simulink model "disturbances_report_sim"  (R2023b)
settings: Solver=ode5  StartTime=0.0  StopTime=5643.69  FixedStep=1  RelTol=1e-3
values from neighbouring files (symbols this model uses):
  A = [0.49 0.49 0.49 0.49 0.49 0.49 0.49 0.49 0.49 0.49 0.49 0.49 0.49 0.49]    [disturbances_report.m]    (also in sat_dist.m = [6*1e-2; 6*1e-2; 6*1e-2; 6*1e-2; 4*1e-2; 4*1e-2; 12*1e-2; 12)
  a = 1 / ( (2/r) - (v^2 / mu) )    [car2par.m]    (also in disturbances_report.m = 6851.22197053)
  c1 = [1 - rho_s; 1 - rho_s; 1 - rho_s]    [disturbances_report.m]
  CD = 2.2    [disturbances_report.m]
  d0 = 1.585*10^-12    (= 1.585e-12)    [disturbances_report.m]
  e = norm(ee)    [car2par.m]    (also in disturbances_report.m = 0.00183012221618)
  H = 60.828    [disturbances_report.m]
  h0 = 450    [disturbances_report.m]
  i = rad2deg(i)    [car2par.m]    (also in disturbances_report.m = 1.69998086203)
  I_ext = diag([I1_ext I2_ext I3_ext])    [disturbances_report.m]
  Iinv_ext = I_ext\eye(3)    [disturbances_report.m]
  jb = [0.01; 0.05; 0.01]    [disturbances_report.m]    (also in sat_dist.m)
  muE = astroConstants(13)    [disturbances_report.m]
  N = [1 0 0]'    [car2par.m]    (also in disturbances_report.m = [0 1 0; 0 -1 0; sqrt(2)/2 0 sqrt(2)/2; -sqrt(2)/2 0 sqrt(2)/; sat_dist.m = [1 0 0; 0 1 0; -1 0 0; 0 -1 0; 0 0 1; 0 0 -1; 1 0 0; -1 0 0;)
  n_sun = sqrt(mu_sun/a_E^3)    [disturbances_report.m]
  nn = sqrt(muE/a^3)    [disturbances_report.m]
  om = rad2deg(om)    [car2par.m]    (also in disturbances_report.m = 1.77284810319)
  OM = rad2deg(OM)    [car2par.m]    (also in disturbances_report.m = 0.55426850949)
  omega0 = zeros(3,1)    [disturbances_report.m]    (also in sat_dist.m = [0; 0; n])
  omegaE = deg2rad(15)/3600    [disturbances_report.m]    (also in sat_dist.m)
  onesM = ones(3, n)    [disturbances_report.m]
  onesV = ones(n,1)    [disturbances_report.m]
  P = astroConstants(31)/(astroConstants(5)*10^3)    [disturbances_report.m]    (also in sat_dist.m = Fe/c)
  r_Fskew = zeros(n*3, n*3)    [disturbances_report.m]
  rho_d = [0.1 0.1 0.1 0.1 0.1 0.1 0.1 0.1 0.1 0.1 0.1 0.1 0.1 0.1]    [disturbances_report.m]
  rho_s = [0.5 0.5 0.5 0.5 0.5 0.5 0.1 0.1 0.1 0.1 0.1 0.1 0.1 0.1]    [disturbances_report.m]
  Rt = astroConstants(23)    [disturbances_report.m]    (also in sat_dist.m)
  s0 = zeros(3,1)    [disturbances_report.m]    (also in sat_dist.m)
  th_0 = 0    [disturbances_report.m]
  tol = 0.2    [disturbances_report.m]
undefined symbols (not defined in the file or in its folder): gh, magnitude
libraries: matrix_library x6, simulink x4, simulink_extras x1, dspmathops x1
(part 1 of 2)
settings Model: Creator=danie  LastModifiedBy=danie

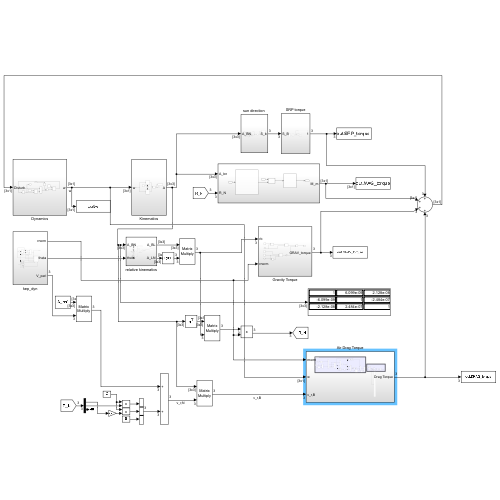
[thumbnail: Simulink's stored preview of the top-level diagram]
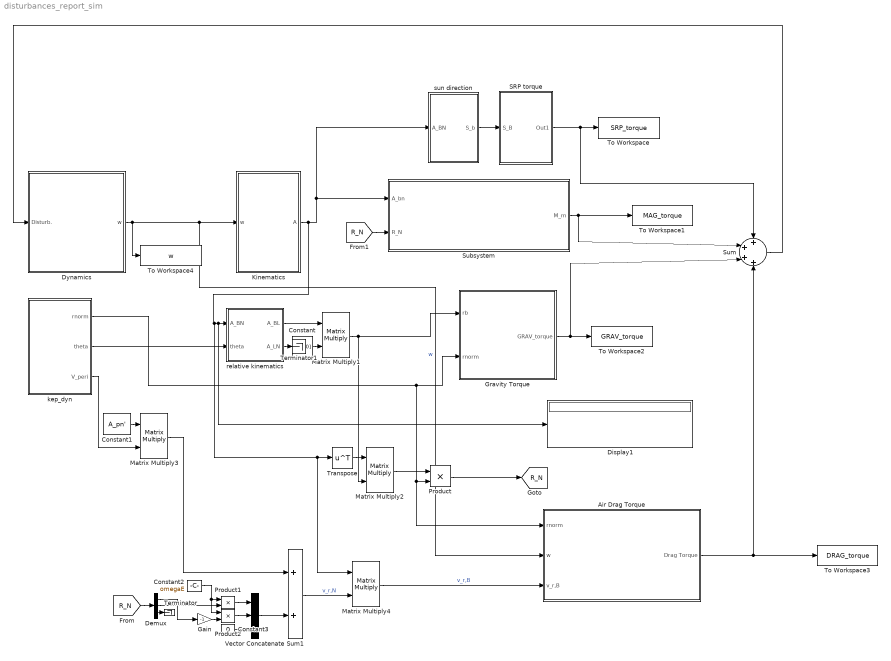
== system disturbances_report_sim ==
  Air Drag Torque : Subsystem
  Constant : Constant  Value=[1;0;0]
  Constant1 : Constant  Value=A_pn'
  Constant2 : Constant  Value=omegaE
  Constant3 : Constant  Value=0
  Demux : Demux  Outputs=3
  Display1 : Display
  Dynamics : Subsystem
  Gain : Gain  Gain=-1
  Gravity Torque : Subsystem
  Kinematics : Subsystem
  Matrix Multiply{1..4} (4 alike) : Product  Multiplication=Matrix(*)
  Product : Product
  Product1 : Product
  Product2 : Product
  SRP torque : Subsystem
  Subsystem : Subsystem
  Sum : Sum  Inputs=++++
  Sum1 : Sum
  Terminator : Terminator
  Terminator1 : Terminator
  To Workspace : ToWorkspace  VariableName=SRP_torque  SaveFormat=Timeseries  SampleTime=-1
  To Workspace1 : ToWorkspace  VariableName=MAG_torque  SampleTime=-1
  To Workspace2 : ToWorkspace  VariableName=GRAV_torque  SaveFormat=Timeseries  SampleTime=-1
  To Workspace3 : ToWorkspace  VariableName=DRAG_torque  SaveFormat=Timeseries  SampleTime=-1
  To Workspace4 : ToWorkspace  VariableName=w  SaveFormat=Timeseries  SampleTime=-1
  Transpose : Math  Operator=transpose
  Vector Concatenate : Concatenate  NumInputs=3
  kep_dyn : Subsystem
  relative kinematics : Subsystem
  "sun direction " : Subsystem
  tag scope: R_N=global
  wires:
  Dynamics/1(w) -> To Workspace4/1, Kinematics/1(w), Air Drag Torque/2(w)  "w"
  kep_dyn/2(theta) -> relative kinematics/2(theta)
  Kinematics/1(A) -> Subsystem/1(A_bn), "sun direction "/1(A_BN), Matrix Multiply4/1, Transpose/1, Display1/1, relative kinematics/1(A_BN)
  SRP torque/1(Out1) -> Sum/1, To Workspace/1
  Matrix Multiply1/1 -> Gravity Torque/1(rb), Matrix Multiply2/2
  Gravity Torque/1(GRAV_torque) -> Sum/3, To Workspace2/1
  relative kinematics/1(A_BL) -> Matrix Multiply1/1
  relative kinematics/2(A_LN) -> Terminator1/1
  "sun direction "/1(S_b) -> SRP torque/1(S_B)
  Sum/1 -> Dynamics/1(Disturb.)
  Constant/1 -> Matrix Multiply1/2
  kep_dyn/1(rnorm) -> Air Drag Torque/1(rnorm), Product/2, Gravity Torque/2(rnorm)
  Transpose/1 -> Matrix Multiply2/1
  Matrix Multiply2/1 -> Product/1
  kep_dyn/3(V_peri) -> Matrix Multiply3/2
  Constant1/1 -> Matrix Multiply3/1
  Matrix Multiply3/1 -> Sum1/1
  Vector Concatenate/1 -> Sum1/2
  Constant3/1 -> Vector Concatenate/3
  Product2/1 -> Vector Concatenate/2
  Product1/1 -> Vector Concatenate/1
  Constant2/1 -> Product2/1, Product1/1
  Product/1 -> [R_N]
  [R_N] -> Demux/1
  Demux/2 -> Product1/2
  Demux/1 -> Gain/1
  Gain/1 -> Product2/2
  Demux/3 -> Terminator/1
  Sum1/1 -> Matrix Multiply4/2  "v_r,N"
  Matrix Multiply4/1 -> Air Drag Torque/3(v_r,B)  "v_r,B"
  Air Drag Torque/1(Drag Torque) -> To Workspace3/1, Sum/4
  [R_N] -> Subsystem/2(R_N)
  Subsystem/1(M_m) -> Sum/2, To Workspace1/1

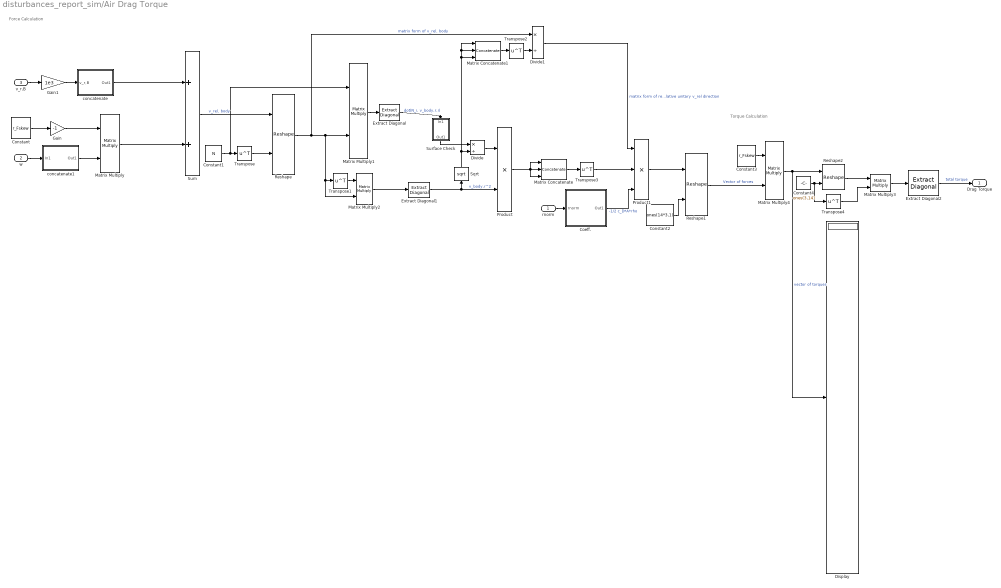
== system disturbances_report_sim/Air Drag Torque ==
  note: Torque Calculation
  note: Force Calculation
  rnorm : Inport
  w : Inport  Port=2
  v_r,B : Inport  Port=3
  Coeff. : Subsystem
  Constant : Constant  Value=r_Fskew
  Constant1 : Constant  Value=N
  Constant2 : Constant  Value=ones(14*3,1)
  Constant3 : Constant  Value=r_Fskew
  Constant4 : Constant  Value=ones(3,14)
  Display : Display
  Divide : Product  Inputs=*/
  Divide1 : Product  Inputs=*/
  Extract Diagonal : matrix_library/Extract Diagonal
      settings: LibrarySourceBlock=|
      | simulink/Matrix
      | Operations/Extract Diagonal
  Extract Diagonal1 : matrix_library/Extract Diagonal
      settings: LibrarySourceBlock=|
      | simulink/Matrix
      | Operations/Extract Diagonal
  Extract Diagonal2 : matrix_library/Extract Diagonal
      settings: LibrarySourceBlock=|
      | simulink/Matrix
      | Operations/Extract Diagonal
  Gain : Gain  Gain=-1
  Gain1 : Gain  Gain=1e3
  Matrix Concatenate : Concatenate  NumInputs=3  Mode=Multidimensional array  ConcatenateDimension=2
  Matrix Concatenate1 : Concatenate  NumInputs=3  Mode=Multidimensional array  ConcatenateDimension=2
  Matrix Multiply{,1..4} (5 alike) : Product  Multiplication=Matrix(*)
  Product : Product
  Product1 : Product  Inputs=3
  Reshape : Reshape  OutputDimensionality=Derive from reference input port
  Reshape1 : Reshape  OutputDimensionality=Derive from reference input port
  Reshape2 : Reshape  OutputDimensionality=Derive from reference input port
  Sqrt : Sqrt
  Sum : Sum
  Surface Check : Subsystem
  Transpose{,1..4} (5 alike) : Math  Operator=transpose
  concatenate : Subsystem
  concatenate1 : Subsystem
  Drag Torque : Outport
  wires:
  Constant/1 -> Gain/1
  Gain/1 -> Matrix Multiply/1
  w/1 -> concatenate1/1(In1)
  concatenate1/1(Out1) -> Matrix Multiply/2
  Matrix Multiply/1 -> Sum/2
  v_r,B/1 -> Gain1/1
  concatenate/1(Out1) -> Sum/1
  Transpose/1 -> Reshape/2
  Constant1/1 -> Matrix Multiply1/1, Transpose/1
  Sum/1 -> Reshape/1  "v_rel, body"
  Reshape/1 -> Transpose1/1, Matrix Multiply2/2, Matrix Multiply1/2, Divide1/1  "matrix form of v_rel, body"
  Matrix Multiply1/1 -> Extract Diagonal/1
  Extract Diagonal/1 -> Surface Check/1(In1)  "dot(N_i, v_body,r,i)"
  Transpose1/1 -> Matrix Multiply2/1
  Matrix Multiply2/1 -> Extract Diagonal1/1
  Extract Diagonal1/1 -> Sqrt/1, Product/2  "v_body,r^2"
  Sqrt/1 -> Divide/2, Matrix Concatenate1/1, Matrix Concatenate1/2, Matrix Concatenate1/3
  Divide/1 -> Product/1
  Product/1 -> Matrix Concatenate/3, Matrix Concatenate/1, Matrix Concatenate/2
  Matrix Concatenate1/1 -> Transpose2/1
  Transpose2/1 -> Divide1/2
  Divide1/1 -> Product1/1  "matrix form of relative unitary v_rel direction"
  Matrix Concatenate/1 -> Transpose3/1
  Surface Check/1(Out1) -> Divide/1
  Coeff./1(Out1) -> Product1/3  "-1/2 c_D*A*rho"
  Transpose3/1 -> Product1/2
  Product1/1 -> Reshape1/1
  Reshape1/1 -> Matrix Multiply4/2  "Vector of forces"
  Constant2/1 -> Reshape1/2
  Constant3/1 -> Matrix Multiply4/1
  Matrix Multiply4/1 -> Display/1, Reshape2/1  "vector of torques"
  rnorm/1 -> Coeff./1(rnorm)
  Constant4/1 -> Transpose4/1, Reshape2/2
  Reshape2/1 -> Matrix Multiply3/1
  Transpose4/1 -> Matrix Multiply3/2
  Matrix Multiply3/1 -> Extract Diagonal2/1
  Extract Diagonal2/1 -> Drag Torque/1  "total torque"
  Gain1/1 -> concatenate/1(v_r,B)

== system disturbances_report_sim/Dynamics ==
  Disturb. : Inport
  Constant : Constant  Value=I_ext
  Constant1 : Constant  Value=Iinv_ext
  Cross Product : matrix_library/Cross Product
  Integrator : Integrator  InitialCondition=omega0
  Product : Product  Multiplication=Matrix(*)
  Product1 : Product  Multiplication=Matrix(*)
  Reshape : Reshape  OutputDimensionality=Column vector (2-D)
  Sum : Sum  Inputs=+-
  w : Outport
  wires:
  Constant/1 -> Product/1
  Integrator/1 -> w/1, Cross Product/1, Product/2  "w"
  Constant1/1 -> Product1/1
  Product/1 -> Cross Product/2
  Product1/1 -> Integrator/1  "wdot"
  Disturb./1 -> Reshape/1
  Sum/1 -> Product1/2
  Cross Product/1 -> Sum/2
  Reshape/1 -> Sum/1

== system disturbances_report_sim/Gravity Torque ==
  rb : Inport
  rnorm : Inport  Port=2
  Constant : Constant  Value=muE
  Constant1 : Constant  Value=I_ext
  Constant3 : Constant  Value=3
  Cross Product : matrix_library/Cross Product
  Divide : Product  Inputs=**/
  Gain : Gain  Gain=-1
  Matrix Multiply : Product  Multiplication=Matrix(*)
  Power : Math  Operator=pow
  Product : Product
  GRAV_torque : Outport
  wires:
  Constant1/1 -> Matrix Multiply/1
  rb/1 -> Matrix Multiply/2, Cross Product/2
  Matrix Multiply/1 -> Cross Product/1
  Constant3/1 -> Power/2, Divide/2
  Power/1 -> Divide/3
  Constant/1 -> Divide/1
  Divide/1 -> Gain/1
  Gain/1 -> Product/2
  Cross Product/1 -> Product/1
  Product/1 -> GRAV_torque/1
  rnorm/1 -> Power/1

== system disturbances_report_sim/Kinematics ==
  w : Inport
  Kinematics 312 : Subsystem
  Kinematics 313 : Subsystem
  Merge : Merge
  NOT : Logic  Operator=NOT  IconShape=distinctive  AllPortsSameDT=off  OutDataTypeStr=boolean
  System switcher : Subsystem
  To Workspace : ToWorkspace  VariableName=A  SaveFormat=Timeseries  SampleTime=-1
  A : Outport
  wires:
  NOT/1 -> Kinematics 313/Enable
  w/1 -> Kinematics 312/1(w), Kinematics 313/1(w)
  System switcher/1(flag) -> Kinematics 312/Enable, NOT/1
  Kinematics 313/1(A) -> Merge/2
  Merge/1 -> A/1, To Workspace/1  "A"
  Kinematics 312/1(A) -> Merge/1

== system disturbances_report_sim/SRP torque ==
  S_B : Inport
  Display : Display
  SRP forces calc : Subsystem
  To Workspace : ToWorkspace  VariableName=SRP_F  SaveFormat=Timeseries  SampleTime=-1
  To Workspace1 : ToWorkspace  VariableName=SRP_T  SaveFormat=Timeseries  SampleTime=-1
  equivalent force system : Subsystem
  Out1 : Outport
  wires:
  equivalent force system/1(Torque) -> Display/1, To Workspace1/1, Out1/1
  equivalent force system/2(Resultant) -> To Workspace/1
  S_B/1 -> SRP forces calc/1(In1)  "SUN DIR."
  SRP forces calc/1(forces) -> equivalent force system/1(Forces)

== system disturbances_report_sim/Subsystem ==
  A_bn : Inport
  R_N : Inport  Port=2
  Magnetic Field : Subsystem
  Magnetic Torque 1 : Subsystem
  Matrix Multiply : Product  Multiplication=Matrix(*)
  M_m : Outport
  wires:
  Magnetic Field/1(B_N) -> Matrix Multiply/2
  Matrix Multiply/1 -> Magnetic Torque 1/1(B_b)
  R_N/1 -> Magnetic Field/1(R_N)
  Magnetic Torque 1/1(M_m) -> M_m/1
  A_bn/1 -> Matrix Multiply/1

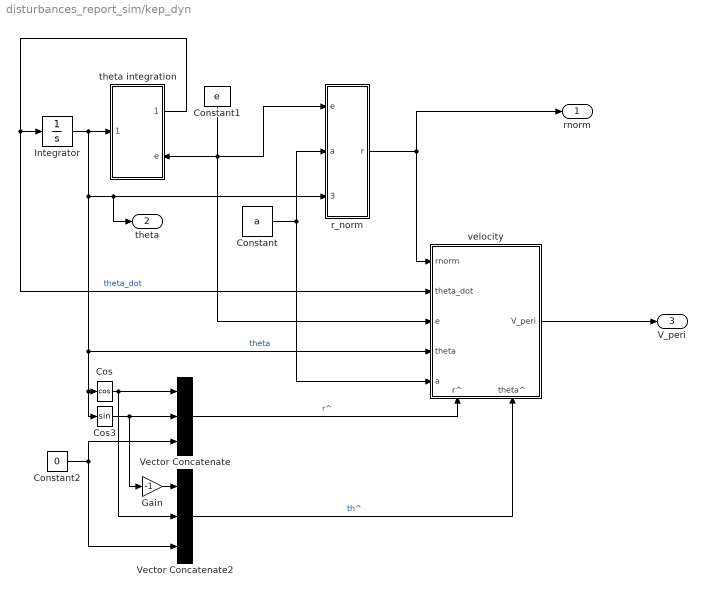
== system disturbances_report_sim/kep_dyn ==
  Constant : Constant  Value=a
  Constant1 : Constant  Value=e
  Constant2 : Constant  Value=0
  Cos : Trigonometry  Operator=cos
  Cos3 : Trigonometry
  Gain : Gain  Gain=-1
  Integrator : Integrator  InitialCondition=th_0
  Vector Concatenate : Concatenate  NumInputs=3
  Vector Concatenate2 : Concatenate  NumInputs=3
  r_norm : Subsystem
  theta integration : Subsystem
      settings: PortSchema="{\"entries\":[{\"content\":{\"sides\":[{\"content\":{\"connectorIds\":[\"In1\"]},\"type\":\"ConnectorPlacement.EquallySpacedRectSide\",\"uuid\":\"3f1b1ec9-07ed-4eb1-9e41-630dc5613e97\"},{\"content\":{\"connectorIds\":[\"Out1\",\"In2\"],\"side\":\"RIGHT\"},\"type\":\"ConnectorPlacement.EquallySpacedRectSide\",\"uuid\":\"22d0f7bc-714c-4365-a26c-07047ff4be14\"},{\"content\":{\"side\":\"TOP\"},\"type\":\"ConnectorPlacement.EquallySpacedRectSide\",\"uuid\":\"875f7006-d698-4730-93ae-1a7d05f24054\"}]},\"type\":\"ConnectorPlacement.EquallySpacedConnector\",\"uuid\":\"799b65b1-faea-432b-9f3f-2d21984184cd\"}],\"packageUris\":[\"http://schema.mathworks.com/mf0/Connector/R2020b\"],\"version\":\"1.0\"}"
  velocity : Subsystem
      settings: PortSchema="{\"entries\":[{\"content\":{\"sides\":[{\"content\":{\"connectorIds\":[\"In1\",\"In2\",\"In3\",\"In4\",\"In5\"]},\"type\":\"ConnectorPlacement.EquallySpacedRectSide\",\"uuid\":\"462ea4ff-c936-4e9a-a15d-c684549947ff\"},{\"content\":{\"connectorIds\":[\"Out1\"],\"side\":\"RIGHT\"},\"type\":\"ConnectorPlacement.EquallySpacedRectSide\",\"uuid\":\"a4e336f6-8704-425f-b778-b72f089cf101\"},{\"content\":{\"side\":\"TOP\"},\"type\":\"ConnectorPlacement.EquallySpacedRectSide\",\"uuid\":\"dc4110a0-1fc3-4f7c-9a82-d4e052a3954d\"},{\"content\":{\"connectorIds\":[\"In6\",\"In7\"],\"side\":\"BOTTOM\"},\"type\":\"ConnectorPlacement.EquallySpacedRectSide\",\"uuid\":\"58c8717a-d2ad-44bd-b5d0-69e581fda9fe\"}]},\"type\":\"ConnectorPlacement.EquallySpacedConnector\",\"uuid\":\"b458c0bc-27e5-4a27-9089-a782da5757b6\"}],\"packageUris\":[\"http://schema.mathworks.com/mf0/Connector/R2020b\"],\"version\":\"1.0\"}"
  rnorm : Outport
  theta : Outport  Port=2
  V_peri : Outport  Port=3
  wires:
  Integrator/1 -> Cos3/1, Cos/1, velocity/4(theta), theta/1, r_norm/3(theta), theta integration/1(theta)  "theta"
  theta integration/1(theta_dot) -> velocity/2(theta_dot), Integrator/1  "theta_dot"
  Constant1/1 -> r_norm/1(e), theta integration/2(e), velocity/3(e)
  r_norm/1(r) -> velocity/1(rnorm), rnorm/1
  Constant/1 -> velocity/5(a), r_norm/2(a)
  Cos/1 -> Vector Concatenate2/2, Vector Concatenate/1
  Cos3/1 -> Gain/1, Vector Concatenate/2
  Constant2/1 -> Vector Concatenate/3, Vector Concatenate2/3
  Gain/1 -> Vector Concatenate2/1
  Vector Concatenate/1 -> velocity/6(r^)  "r^"
  Vector Concatenate2/1 -> velocity/7(theta^)  "th^"
  velocity/1(V_peri) -> V_peri/1

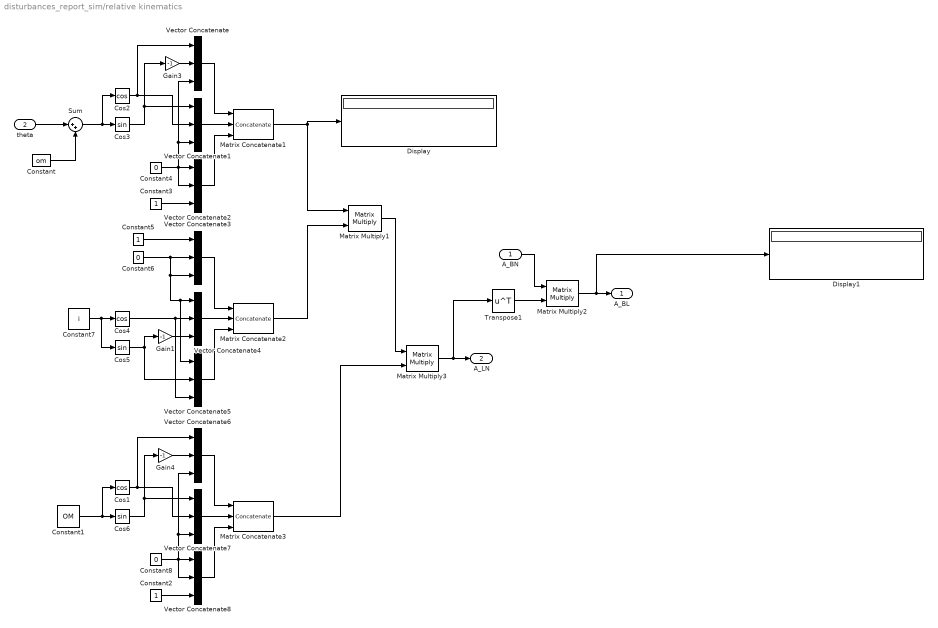
== system disturbances_report_sim/relative kinematics ==
  A_BN : Inport
  theta : Inport  Port=2
  Constant : Constant  Value=om
  Constant1 : Constant  Value=OM
  Constant2 : Constant
  Constant3 : Constant
  Constant4 : Constant  Value=0
  Constant5 : Constant
  Constant6 : Constant  Value=0
  Constant7 : Constant  Value=i
  Constant8 : Constant  Value=0
  Cos1 : Trigonometry  Operator=cos
  Cos2 : Trigonometry  Operator=cos
  Cos3 : Trigonometry
  Cos4 : Trigonometry  Operator=cos
  Cos5 : Trigonometry
  Cos6 : Trigonometry
  Display : Display
  Display1 : Display
  Gain1 : Gain  Gain=-1
  Gain3 : Gain  Gain=-1
  Gain4 : Gain  Gain=-1
  Matrix Concatenate1 : Concatenate  NumInputs=3  Mode=Multidimensional array  ConcatenateDimension=2
  Matrix Concatenate2 : Concatenate  NumInputs=3  Mode=Multidimensional array  ConcatenateDimension=2
  Matrix Concatenate3 : Concatenate  NumInputs=3  Mode=Multidimensional array  ConcatenateDimension=2
  Matrix Multiply1 : Product  Multiplication=Matrix(*)
  Matrix Multiply2 : Product  Multiplication=Matrix(*)
  Matrix Multiply3 : Product  Multiplication=Matrix(*)
  Sum : Sum  Inputs=|++
  Transpose1 : Math  Operator=transpose
  Vector Concatenate{,1..8} (9 alike) : Concatenate  NumInputs=3
  A_BL : Outport
  A_LN : Outport  Port=2
  wires:
  Cos2/1 -> Vector Concatenate1/2, Vector Concatenate/1
  Constant4/1 -> Vector Concatenate2/2, Vector Concatenate/3, Vector Concatenate1/3, Vector Concatenate2/1
  Constant3/1 -> Vector Concatenate2/3
  Cos3/1 -> Vector Concatenate1/1, Gain3/1
  Vector Concatenate/1 -> Matrix Concatenate1/1
  Vector Concatenate1/1 -> Matrix Concatenate1/2
  Vector Concatenate2/1 -> Matrix Concatenate1/3
  Vector Concatenate5/1 -> Matrix Concatenate2/3
  Constant7/1 -> Cos4/1, Cos5/1
  Vector Concatenate3/1 -> Matrix Concatenate2/1
  Vector Concatenate4/1 -> Matrix Concatenate2/2
  Constant5/1 -> Vector Concatenate3/1
  Constant6/1 -> Vector Concatenate5/1, Vector Concatenate4/1, Vector Concatenate3/3, Vector Concatenate3/2
  Cos4/1 -> Vector Concatenate4/2, Vector Concatenate5/3
  Cos5/1 -> Vector Concatenate5/2, Gain1/1
  Matrix Concatenate1/1 -> Matrix Multiply1/1, Display/1
  Matrix Concatenate2/1 -> Matrix Multiply1/2
  Matrix Multiply1/1 -> Matrix Multiply3/1
  A_BN/1 -> Matrix Multiply2/1
  Transpose1/1 -> Matrix Multiply2/2
  Matrix Multiply2/1 -> Display1/1, A_BL/1
  Constant/1 -> Sum/2
  theta/1 -> Sum/1
  Sum/1 -> Cos2/1, Cos3/1
  Constant8/1 -> Vector Concatenate8/2, Vector Concatenate6/3, Vector Concatenate7/3, Vector Concatenate8/1
  Vector Concatenate7/1 -> Matrix Concatenate3/2
  Vector Concatenate6/1 -> Matrix Concatenate3/1
  Vector Concatenate8/1 -> Matrix Concatenate3/3
  Matrix Concatenate3/1 -> Matrix Multiply3/2
  Cos1/1 -> Vector Concatenate7/2, Vector Concatenate6/1
  Constant2/1 -> Vector Concatenate8/3
  Cos6/1 -> Vector Concatenate7/1, Gain4/1
  Constant1/1 -> Cos1/1, Cos6/1
  Matrix Multiply3/1 -> Transpose1/1, A_LN/1
  Gain3/1 -> Vector Concatenate/2
  Gain4/1 -> Vector Concatenate6/2
  Gain1/1 -> Vector Concatenate4/3

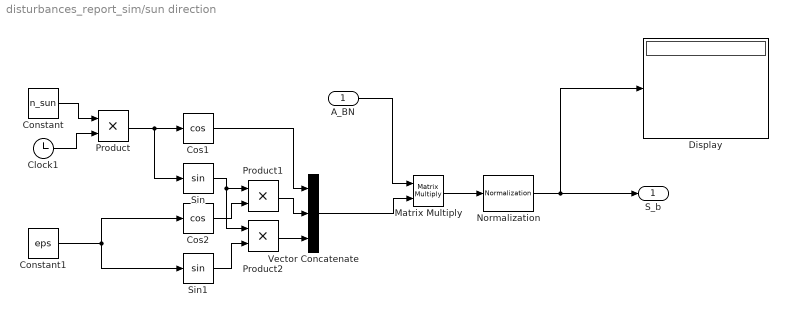
== system disturbances_report_sim/sun direction  ==
  A_BN : Inport
  Clock1 : Clock
  Constant : Constant  Value=n_sun
  Constant1 : Constant  Value=eps
  Cos1 : Trigonometry  Operator=cos
  Cos2 : Trigonometry  Operator=cos
  Display : Display
  Matrix Multiply : Product  Multiplication=Matrix(*)
  Normalization : dspmathops/Normalization  NormType=Squared 2-norm  Bias=1e-10  NormOver=Each column  Dimension=1  roundingMode=Floor  overflowMode=off  accumDataTypeStr=Inherit: Same as product output  accumLastDataTypeStr=Inherit: Same as product output  outputDataTypeStr=Inherit: Same as product output  outputMin=[]  outputMax=[]  outputLastDataTypeStr=Inherit: Same as product output
  Product : Product
  Product1 : Product
  Product2 : Product
  Sin : Trigonometry
  Sin1 : Trigonometry
  Vector Concatenate : Concatenate  NumInputs=3
  S_b : Outport
  wires:
  Constant/1 -> Product/1
  Clock1/1 -> Product/2
  Product/1 -> Sin/1, Cos1/1
  Constant1/1 -> Sin1/1, Cos2/1
  Sin/1 -> Product2/1, Product1/1
  Cos2/1 -> Product1/2
  Sin1/1 -> Product2/2
  Cos1/1 -> Vector Concatenate/1
  Product1/1 -> Vector Concatenate/2
  Product2/1 -> Vector Concatenate/3
  Matrix Multiply/1 -> Normalization/1
  A_BN/1 -> Matrix Multiply/1
  Normalization/1 -> Display/1, S_b/1
  Vector Concatenate/1 -> Matrix Multiply/2

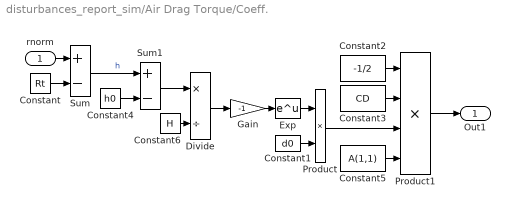
== system disturbances_report_sim/Air Drag Torque/Coeff. ==
  rnorm : Inport
  Constant : Constant  Value=Rt
  Constant1 : Constant  Value=d0
  Constant2 : Constant  Value=-1/2
  Constant3 : Constant  Value=CD
  Constant4 : Constant  Value=h0
  Constant5 : Constant  Value=A(1,1)
  Constant6 : Constant  Value=H
  Divide : Product  Inputs=*/
  Exp : Math
  Gain : Gain  Gain=-1
  Product : Product
  Product1 : Product  Inputs=4
  Sum : Sum  Inputs=+-
  Sum1 : Sum  Inputs=+-
  Out1 : Outport
  wires:
  Constant2/1 -> Product1/1
  Constant5/1 -> Product1/4
  Product1/1 -> Out1/1
  Constant3/1 -> Product1/2
  Sum/1 -> Sum1/1  "h"
  rnorm/1 -> Sum/1
  Constant/1 -> Sum/2
  Constant4/1 -> Sum1/2
  Divide/1 -> Gain/1
  Sum1/1 -> Divide/1
  Constant6/1 -> Divide/2
  Gain/1 -> Exp/1
  Exp/1 -> Product/1
  Constant1/1 -> Product/2
  Product/1 -> Product1/3

== system disturbances_report_sim/Air Drag Torque/Surface Check ==
  In1 : Inport
  Compare To Constant : simulink/Logic and Bit Operations/Compare To Constant  relop=>  const=0  OutDataTypeStr=boolean
  Product5 : Product
  Out1 : Outport
  wires:
  Product5/1 -> Out1/1
  Compare To Constant/1 -> Product5/2
  In1/1 -> Compare To Constant/1, Product5/1

== system disturbances_report_sim/Air Drag Torque/concatenate ==
  v_r,B : Inport
  Vector Concatenate : Concatenate  NumInputs=14
  Out1 : Outport
  wires:
  Vector Concatenate/1 -> Out1/1
  v_r,B/1 -> Vector Concatenate/1, Vector Concatenate/2, Vector Concatenate/3, Vector Concatenate/4, Vector Concatenate/5, Vector Concatenate/6, Vector Concatenate/7, Vector Concatenate/8, Vector Concatenate/9, Vector Concatenate/10, Vector Concatenate/11, Vector Concatenate/12, Vector Concatenate/13, Vector Concatenate/14

== system disturbances_report_sim/Air Drag Torque/concatenate1 ==
  In1 : Inport
  Vector Concatenate : Concatenate  NumInputs=14
  Out1 : Outport
  wires:
  In1/1 -> Vector Concatenate/14, Vector Concatenate/13, Vector Concatenate/12, Vector Concatenate/11, Vector Concatenate/10, Vector Concatenate/9, Vector Concatenate/8, Vector Concatenate/7, Vector Concatenate/6, Vector Concatenate/5, Vector Concatenate/4, Vector Concatenate/3, Vector Concatenate/2, Vector Concatenate/1
  Vector Concatenate/1 -> Out1/1

== system disturbances_report_sim/Kinematics/Kinematics 312 ==
  w : Inport
  Enable : EnablePort  StatesWhenEnabling=reset
  A - s_312 : Subsystem
  Euler angles : Subsystem
  IC : InitialCondition  Value=s0
  s_312 - A : Subsystem
  s_313 - A : Subsystem
  A : Outport
  wires:
  s_312 - A/1(A) -> A/1  "A"
  Euler angles/1(s) -> s_312 - A/1(s)  "s"
  w/1 -> Euler angles/1(w)
  IC/1 -> Euler angles/2(s0)
  A - s_312/1(s) -> IC/1
  s_313 - A/1(A) -> A - s_312/1(A)
  [s_313] -> s_313 - A/1(s)

== system disturbances_report_sim/Kinematics/Kinematics 313 ==
  w : Inport
  Enable : EnablePort  StatesWhenEnabling=reset
  A - s_313 : Subsystem
  Euler angles : Subsystem
  s_312 - A : Subsystem
  s_313 - A : Subsystem
  A : Outport
  wires:
  w/1 -> Euler angles/1(w)
  Euler angles/1(s) -> s_313 - A/1(s)
  s_313 - A/1(A) -> A/1
  A - s_313/1(s) -> Euler angles/2(s0)
  s_312 - A/1(A) -> A - s_313/1(A)
  [s_312] -> s_312 - A/1(s)

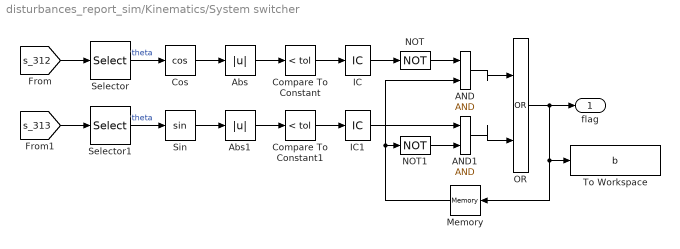
== system disturbances_report_sim/Kinematics/System switcher ==
  AND : Logic  IconShape=distinctive  AllPortsSameDT=off  OutDataTypeStr=boolean
  AND1 : Logic  IconShape=distinctive  AllPortsSameDT=off  OutDataTypeStr=boolean
  Abs : Abs  SaturateOnIntegerOverflow=off
  Abs1 : Abs  SaturateOnIntegerOverflow=off
  Compare To Constant : simulink/Logic and Bit Operations/Compare To Constant  relop=<  const=tol  OutDataTypeStr=boolean
  Compare To Constant1 : simulink/Logic and Bit Operations/Compare To Constant  relop=<  const=tol  OutDataTypeStr=boolean
  Cos : Trigonometry  Operator=cos
  IC : InitialCondition  Value=0
  IC1 : InitialCondition  Value=0
  Memory : Memory  InitialCondition=1
  NOT : Logic  Operator=NOT  IconShape=distinctive  AllPortsSameDT=off  OutDataTypeStr=boolean
  NOT1 : Logic  Operator=NOT  IconShape=distinctive  AllPortsSameDT=off  OutDataTypeStr=boolean
  OR : Logic  Operator=OR  IconShape=distinctive  AllPortsSameDT=off  OutDataTypeStr=boolean
  Selector : Selector  InputPortWidth=3  IndexOptions=Index vector (dialog)  Indices=2  OutputSizes=1
  Selector1 : Selector  InputPortWidth=3  IndexOptions=Index vector (dialog)  Indices=2  OutputSizes=1
  Sin : Trigonometry
  To Workspace : ToWorkspace  VariableName=b  SaveFormat=Timeseries  SampleTime=-1
  flag : Outport
  wires:
  Cos/1 -> Abs/1
  [s_312] -> Selector/1
  Compare To Constant/1 -> IC/1
  Selector1/1 -> Sin/1  "theta"
  Abs/1 -> Compare To Constant/1
  Compare To Constant1/1 -> IC1/1
  Selector/1 -> Cos/1  "theta"
  Abs1/1 -> Compare To Constant1/1
  Sin/1 -> Abs1/1
  [s_313] -> Selector1/1
  IC/1 -> NOT/1
  NOT/1 -> AND/1
  AND/1 -> OR/1
  NOT1/1 -> AND1/2
  IC1/1 -> AND1/1
  AND1/1 -> OR/2
  OR/1 -> To Workspace/1, Memory/1, flag/1
  Memory/1 -> AND/2, NOT1/1

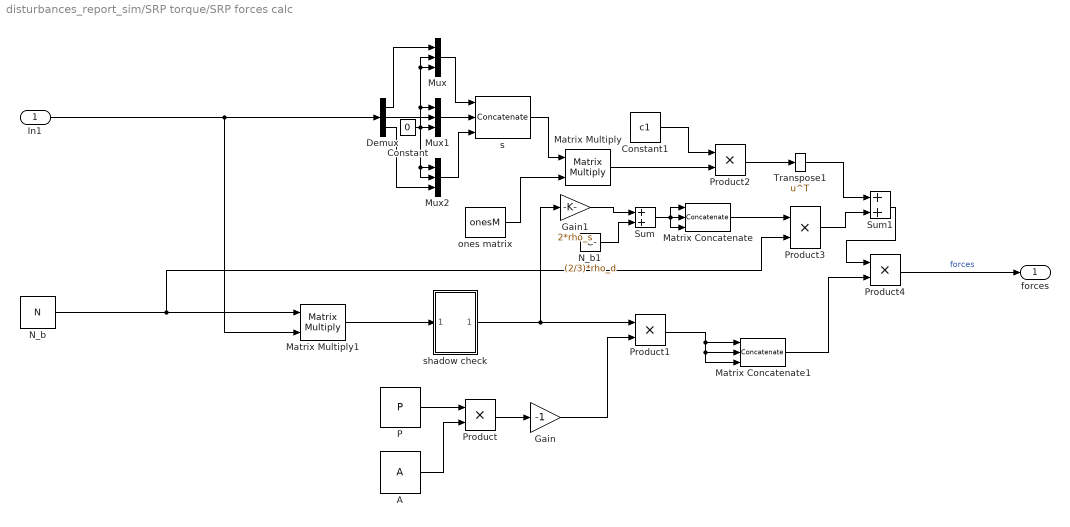
== system disturbances_report_sim/SRP torque/SRP forces calc ==
  In1 : Inport
  A : Constant  Value=A
  Constant : Constant  Value=0
  Constant1 : Constant  Value=c1
  Demux : Demux  Outputs=3
  Gain : Gain  Gain=-1
  Gain1 : Gain  Gain=2*rho_s
  Matrix Concatenate : Concatenate  NumInputs=3  Mode=Multidimensional array  ConcatenateDimension=2
  Matrix Concatenate1 : Concatenate  NumInputs=3  Mode=Multidimensional array  ConcatenateDimension=2
  Matrix Multiply : Product  Multiplication=Matrix(*)
  Matrix Multiply1 : Product  Multiplication=Matrix(*)
  Mux : Mux  Inputs=3
  Mux1 : Mux  Inputs=3
  Mux2 : Mux  Inputs=3
  N_b : Constant  Value=N
  N_b1 : Constant  Value=(2/3)*rho_d
  P : Constant  Value=P
  Product{,1..4} (5 alike) : Product
  Sum : Sum
  Sum1 : Sum
  Transpose1 : Math  Operator=transpose
  ones matrix : Constant  Value=onesM
  "s " : Concatenate  NumInputs=3  Mode=Multidimensional array  ConcatenateDimension=2
  shadow check : Subsystem
  forces : Outport
  wires:
  Product2/1 -> Transpose1/1
  Matrix Multiply/1 -> Product2/2
  N_b/1 -> Product3/2, Matrix Multiply1/1
  P/1 -> Product/1
  ones matrix/1 -> Matrix Multiply/2
  Mux/1 -> "s "/1
  Sum1/1 -> Product4/1
  Mux2/1 -> "s "/3
  Matrix Multiply1/1 -> shadow check/1(In1)
  Gain1/1 -> Sum/1
  Constant/1 -> Mux2/2, Mux2/1, Mux/2, Mux/3, Mux1/1, Mux1/3
  Demux/1 -> Mux/1
  N_b1/1 -> Sum/2
  Product3/1 -> Sum1/2
  Demux/3 -> Mux2/3
  Product1/1 -> Matrix Concatenate1/3, Matrix Concatenate1/2, Matrix Concatenate1/1
  In1/1 -> Demux/1, Matrix Multiply1/2
  Product/1 -> Gain/1
  Matrix Concatenate/1 -> Product3/1
  A/1 -> Product/2
  shadow check/1(Out1) -> Product1/1, Gain1/1
  Demux/2 -> Mux1/2
  Mux1/1 -> "s "/2
  Sum/1 -> Matrix Concatenate/3, Matrix Concatenate/1, Matrix Concatenate/2
  Gain/1 -> Product1/2
  Matrix Concatenate1/1 -> Product4/2
  "s "/1 -> Matrix Multiply/1
  Transpose1/1 -> Sum1/1
  Constant1/1 -> Product2/1
  Product4/1 -> forces/1  "forces"

== system disturbances_report_sim/SRP torque/equivalent force system ==
  Forces : Inport
  Constant : Constant  Value=r_Fskew
  Constant1 : Constant  Value=onesV
  Display1 : Display
  Display2 : Display
  Matrix Multiply : Product  Multiplication=Matrix(*)
  Matrix Multiply1 : Product  Multiplication=Matrix(*)
  Matrix Multiply2 : Product  Multiplication=Matrix(*)
  Reshape : Reshape  OutputDimensionality=Column vector (2-D)
  Reshape1 : Reshape  OutputDimensionality=Derive from reference input port
  Transpose : Math  Operator=transpose
  Torque : Outport
  Resultant : Outport  Port=2
  wires:
  Forces/1 -> Transpose/1
  Reshape/1 -> Display2/1, Matrix Multiply/2
  Constant/1 -> Matrix Multiply/1
  Transpose/1 -> Reshape/1, Matrix Multiply2/1, Reshape1/2
  Matrix Multiply/1 -> Reshape1/1
  Matrix Multiply1/1 -> Display1/1, Torque/1
  Reshape1/1 -> Matrix Multiply1/1
  Constant1/1 -> Matrix Multiply1/2, Matrix Multiply2/2
  Matrix Multiply2/1 -> Resultant/1

== system disturbances_report_sim/Subsystem/Magnetic Field ==
  R_N : Inport
  Cartesian to Spherical : simulink_extras/Transformations/Cartesian to Spherical
  Constant : Constant  Value=gh
  Demux : Demux  Outputs=3
  MATLAB Function : MATLAB Function  TreatAsAtomicUnit=on
  Matrix Multiply : Product  Multiplication=Matrix(*)
  Matrix Multiply1 : Product  Multiplication=Matrix(*)
  R_en : Subsystem
  Transpose : Math  Operator=transpose
  B_N : Outport
  wires:
  R_en/1(R_en) -> Transpose/1, Matrix Multiply/1
  Demux/1 -> Cartesian to Spherical/1
  Demux/2 -> Cartesian to Spherical/2
  Demux/3 -> Cartesian to Spherical/3
  Matrix Multiply/1 -> Demux/1
  Cartesian to Spherical/1 -> MATLAB Function/1(r)
  Cartesian to Spherical/2 -> MATLAB Function/2(theta)
  Cartesian to Spherical/3 -> MATLAB Function/3(phi)
  Transpose/1 -> Matrix Multiply1/1
  MATLAB Function/1(B) -> Matrix Multiply1/2
  Constant/1 -> MATLAB Function/4(gh)
  R_N/1 -> Matrix Multiply/2
  Matrix Multiply1/1 -> B_N/1

== system disturbances_report_sim/Subsystem/Magnetic Torque 1 ==
  B_b : Inport
  Constant3 : Constant  Value=jb
  Cross Product : matrix_library/Cross Product
  M_m : Outport
  wires:
  Cross Product/1 -> M_m/1
  Constant3/1 -> Cross Product/1
  B_b/1 -> Cross Product/2

== system disturbances_report_sim/kep_dyn/r_norm ==
  e : Inport
  a : Inport  Port=2
  theta : Inport  Port=3
  Constant1 : Constant
  Cos : Trigonometry  Operator=cos
  Divide : Product  Inputs=*/
  Power : Math  Operator=magnitude^2
  Product : Product
  Product1 : Product
  Sum : Sum  Inputs=+-
  Sum2 : Sum
  r : Outport
  wires:
  e/1 -> Product1/2, Power/1
  Power/1 -> Sum/2
  Constant1/1 -> Sum2/2, Sum/1
  Sum/1 -> Product/2
  a/1 -> Product/1
  theta/1 -> Cos/1
  Cos/1 -> Product1/1
  Product1/1 -> Sum2/1
  Divide/1 -> r/1
  Sum2/1 -> Divide/2
  Product/1 -> Divide/1

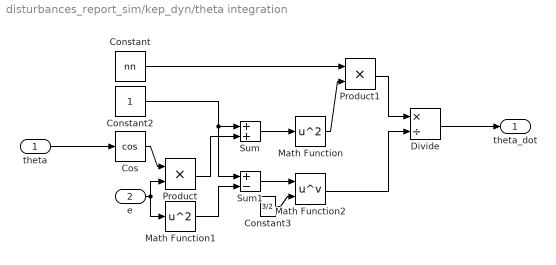
== system disturbances_report_sim/kep_dyn/theta integration ==
  theta : Inport
  e : Inport  Port=2
  Constant : Constant  Value=nn
  Constant2 : Constant
  Constant3 : Constant  Value=3/2
  Cos : Trigonometry  Operator=cos
  Divide : Product  Inputs=*/
  Math Function : Math  Operator=square
  Math Function1 : Math  Operator=square
  Math Function2 : Math  Operator=pow
  Product : Product
  Product1 : Product
  Sum : Sum
  Sum1 : Sum  Inputs=+-
  theta_dot : Outport
  wires:
  Product1/1 -> Divide/1
  Product/1 -> Sum/2
  Math Function2/1 -> Divide/2
  Sum1/1 -> Math Function2/1
  Constant2/1 -> Sum1/1, Sum/1
  Math Function1/1 -> Sum1/2
  e/1 -> Product/2, Math Function1/1
  Constant3/1 -> Math Function2/2
  Constant/1 -> Product1/1
  Sum/1 -> Math Function/1
  Math Function/1 -> Product1/2
  Cos/1 -> Product/1
  theta/1 -> Cos/1
  Divide/1 -> theta_dot/1

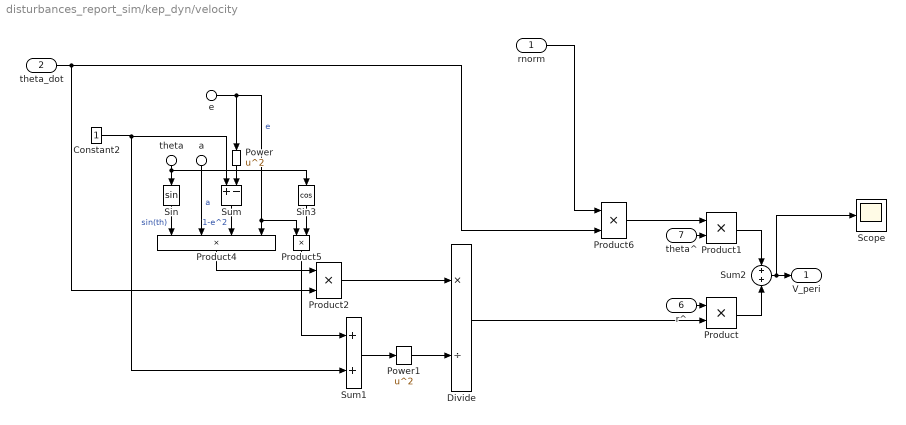
== system disturbances_report_sim/kep_dyn/velocity ==
  rnorm : Inport
  theta_dot : Inport  Port=2
  e : Inport  Port=3
  theta : Inport  Port=4
  a : Inport  Port=5
  r^ : Inport  Port=6
  theta^ : Inport  Port=7
  Constant2 : Constant
  Divide : Product  Inputs=*/
  Power : Math  Operator=square
  Power1 : Math  Operator=square
  Product{,1..2,5..6} (5 alike) : Product
  Product4 : Product  Inputs=4
  Scope : Scope
  Sin : Trigonometry
  Sin3 : Trigonometry  Operator=cos
  Sum : Sum  Inputs=+-
  Sum1 : Sum
  Sum2 : Sum
  V_peri : Outport
  wires:
  Product2/1 -> Divide/1
  Product6/1 -> Product1/1
  theta/1 -> Sin3/1, Sin/1
  Constant2/1 -> Sum1/2, Sum/1
  Sin/1 -> Product4/1  "sin(th)"
  Power1/1 -> Divide/2
  Product4/1 -> Product2/1
  Divide/1 -> Product/2
  Sum/1 -> Product4/3  "1-e^2"
  theta_dot/1 -> Product2/2, Product6/2
  Sum1/1 -> Power1/1
  Power/1 -> Sum/2
  a/1 -> Product4/2  "a"
  rnorm/1 -> Product6/1
  e/1 -> Power/1, Product5/1, Product4/4  "e"
  Sin3/1 -> Product5/2
  Product5/1 -> Sum1/1
  r^/1 -> Product/1
  theta^/1 -> Product1/2
  Sum2/1 -> Scope/1, V_peri/1
  Product1/1 -> Sum2/1
  Product/1 -> Sum2/2

== system disturbances_report_sim/Kinematics/Kinematics 312/A - s_312 ==
  A : Inport
  Asin : Trigonometry  Operator=asin
  Atan1 : Trigonometry  Operator=atan2
  Atan2 : Trigonometry  Operator=atan2
  Gain : Gain  Gain=-1
  Gain1 : Gain  Gain=-1
  Mux : Mux  Inputs=3
  Selector : Selector  NumberOfDimensions=2  InputPortWidth=3  IndexOptions=Index vector (dialog),Index vector (dialog)  Indices=2,1  OutputSizes=1,1
  Selector1 : Selector  NumberOfDimensions=2  InputPortWidth=3  IndexOptions=Index vector (dialog),Index vector (dialog)  Indices=2,2  OutputSizes=1,1
  Selector2 : Selector  NumberOfDimensions=2  InputPortWidth=3  IndexOptions=Index vector (dialog),Index vector (dialog)  Indices=2,3  OutputSizes=1,1
  Selector3 : Selector  NumberOfDimensions=2  InputPortWidth=3  IndexOptions=Index vector (dialog),Index vector (dialog)  Indices=1,3  OutputSizes=1,1
  Selector4 : Selector  NumberOfDimensions=2  InputPortWidth=3  IndexOptions=Index vector (dialog),Index vector (dialog)  Indices=3,3  OutputSizes=1,1
  s : Outport
  wires:
  Mux/1 -> s/1
  Selector4/1 -> Atan1/2  "a33"
  Atan1/1 -> Mux/3  "psi"
  Atan2/1 -> Mux/1  "phi"
  A/1 -> Selector2/1, Selector1/1, Selector/1, Selector3/1, Selector4/1
  Selector2/1 -> Asin/1  "a23"
  Selector3/1 -> Gain1/1  "a13"
  Selector1/1 -> Atan2/2  "a22"
  Selector/1 -> Gain/1  "a21"
  Asin/1 -> Mux/2  "theta"
  Gain/1 -> Atan2/1
  Gain1/1 -> Atan1/1

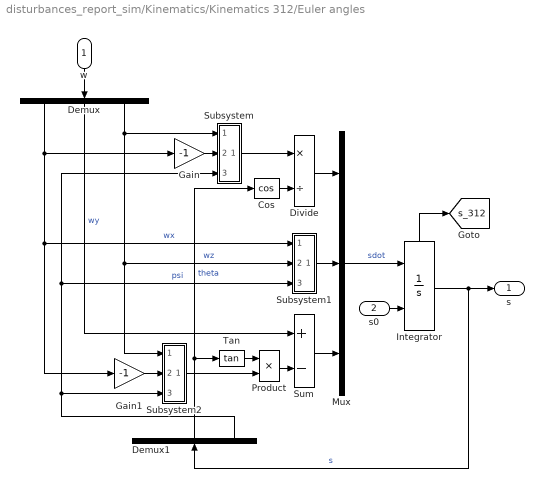
== system disturbances_report_sim/Kinematics/Kinematics 312/Euler angles ==
  w : Inport
  s0 : Inport  Port=2
  Cos : Trigonometry  Operator=cos
  Demux : Demux  Outputs=3
  Demux1 : Demux  Outputs=3
  Divide : Product  Inputs=*/
  Gain : Gain  Gain=-1
  Gain1 : Gain  Gain=-1
  Integrator : Integrator  InitialConditionSource=external  InitialCondition=s0  WrapState=on  WrappedStateUpperValue=2*pi  WrappedStateLowerValue=0  ShowStatePort=on
  Mux : Mux  Inputs=3
  Product : Product
  Subsystem : Subsystem
  Subsystem1 : Subsystem
  Subsystem2 : Subsystem
  Sum : Sum  Inputs=+-
  Tan : Trigonometry  Operator=tan
  s : Outport
  tag scope: s_312=global
  wires:
  w/1 -> Demux/1
  Integrator/1 -> Demux1/1, s/1  "s"
  Demux/3 -> Subsystem2/1(In1), Subsystem1/2(In2), Subsystem/1(In1)  "wz"
  Gain/1 -> Subsystem/2(In2)
  Demux/1 -> Gain1/1, Subsystem1/1(In1), Gain/1  "wx"
  Demux1/3 -> Subsystem2/3(In3), Subsystem1/3(In3), Subsystem/3(In3)  "psi"
  Subsystem/1(Out1) -> Divide/1
  Cos/1 -> Divide/2
  Demux1/2 -> Cos/1, Tan/1  "theta"
  Divide/1 -> Mux/1
  Subsystem1/1(Out1) -> Mux/2
  Gain1/1 -> Subsystem2/2(In2)
  Tan/1 -> Product/1
  Subsystem2/1(Out1) -> Product/2
  Product/1 -> Sum/2
  Demux/2 -> Sum/1  "wy"
  Sum/1 -> Mux/3
  Mux/1 -> Integrator/1  "sdot"
  s0/1 -> Integrator/2
  Integrator/State -> [s_312]

== system disturbances_report_sim/Kinematics/Kinematics 312/s_312 - A ==
  s : Inport
  Demux : Demux  Outputs=3
  Product : Product  Inputs=3  Multiplication=Matrix(*)
  R1 : Subsystem
  R2 : Subsystem
  R3 : Subsystem
  A : Outport
  wires:
  s/1 -> Demux/1  "s"
  R1/1(R1) -> Product/2
  R3/1(R3) -> Product/3
  R2/1(R2) -> Product/1
  Product/1 -> A/1
  Demux/2 -> R1/1(x)  "theta"
  Demux/1 -> R3/1(x)  "phi"
  Demux/3 -> R2/1(x)  "psi"

== system disturbances_report_sim/Kinematics/Kinematics 312/s_313 - A ==
  s : Inport
  Demux : Demux  Outputs=3
  Product : Product  Inputs=3  Multiplication=Matrix(*)
  R1 : Subsystem
  R3_1 : Subsystem
  R3_2 : Subsystem
  A : Outport
  wires:
  Demux/3 -> R3_2/1(x)  "psi"
  Demux/1 -> R3_1/1(x)  "phi"
  Demux/2 -> R1/1(x)  "theta"
  Product/1 -> A/1
  R1/1(R1) -> Product/2
  s/1 -> Demux/1  "s"
  R3_1/1(R3) -> Product/3
  R3_2/1(R3) -> Product/1

== system disturbances_report_sim/Kinematics/Kinematics 313/A - s_313 ==
  A : Inport
  Acos : Trigonometry  Operator=acos
  Atan1 : Trigonometry  Operator=atan2
  Atan2 : Trigonometry  Operator=atan2
  Gain : Gain  Gain=-1
  Mux : Mux  Inputs=3
  Selector : Selector  NumberOfDimensions=2  InputPortWidth=3  IndexOptions=Index vector (dialog),Index vector (dialog)  Indices=3,1  OutputSizes=1,1
  Selector1 : Selector  NumberOfDimensions=2  InputPortWidth=3  IndexOptions=Index vector (dialog),Index vector (dialog)  Indices=3,2  OutputSizes=1,1
  Selector2 : Selector  NumberOfDimensions=2  InputPortWidth=3  IndexOptions=Index vector (dialog),Index vector (dialog)  Indices=3,3  OutputSizes=1,1
  Selector3 : Selector  NumberOfDimensions=2  InputPortWidth=3  IndexOptions=Index vector (dialog),Index vector (dialog)  Indices=1,3  OutputSizes=1,1
  Selector4 : Selector  NumberOfDimensions=2  InputPortWidth=3  IndexOptions=Index vector (dialog),Index vector (dialog)  Indices=2,3  OutputSizes=1,1
  s : Outport
  wires:
  Acos/1 -> Mux/2  "theta"
  Selector/1 -> Atan2/1  "a31"
  Selector1/1 -> Gain/1  "a32"
  Selector3/1 -> Atan1/1  "a13"
  Selector2/1 -> Acos/1  "a33"
  A/1 -> Selector4/1, Selector3/1, Selector/1, Selector1/1, Selector2/1
  Atan2/1 -> Mux/1  "phi"
  Atan1/1 -> Mux/3  "psi"
  Gain/1 -> Atan2/2
  Selector4/1 -> Atan1/2  "a23"
  Mux/1 -> s/1

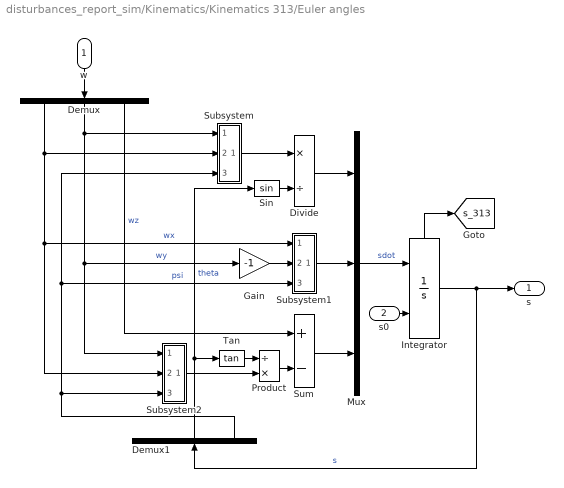
== system disturbances_report_sim/Kinematics/Kinematics 313/Euler angles ==
  w : Inport
  s0 : Inport  Port=2
  Demux : Demux  Outputs=3
  Demux1 : Demux  Outputs=3
  Divide : Product  Inputs=*/
  Gain : Gain  Gain=-1
  Integrator : Integrator  InitialConditionSource=external  InitialCondition=s0  WrapState=on  WrappedStateUpperValue=2*pi  WrappedStateLowerValue=0  ShowStatePort=on
  Mux : Mux  Inputs=3
  Product : Product  Inputs=/*
  Sin : Trigonometry
  Subsystem : Subsystem
  Subsystem1 : Subsystem
  Subsystem2 : Subsystem
  Sum : Sum  Inputs=+-
  Tan : Trigonometry  Operator=tan
  s : Outport
  tag scope: s_313=global
  wires:
  Mux/1 -> Integrator/1  "sdot"
  Sum/1 -> Mux/3
  Demux/2 -> Subsystem/1(In1), Subsystem2/1(In1), Gain/1  "wy"
  Product/1 -> Sum/2
  Subsystem2/1(Out1) -> Product/2
  Tan/1 -> Product/1
  Subsystem1/1(Out1) -> Mux/2
  Divide/1 -> Mux/1
  Demux1/2 -> Sin/1, Tan/1  "theta"
  Subsystem/1(Out1) -> Divide/1
  Demux1/3 -> Subsystem/3(In3), Subsystem1/3(In3), Subsystem2/3(In3)  "psi"
  Demux/1 -> Subsystem2/2(In2), Subsystem1/1(In1), Subsystem/2(In2)  "wx"
  Demux/3 -> Sum/1  "wz"
  Integrator/1 -> Demux1/1, s/1  "s"
  w/1 -> Demux/1
  Sin/1 -> Divide/2
  Gain/1 -> Subsystem1/2(In2)
  s0/1 -> Integrator/2
  Integrator/State -> [s_313]

== system disturbances_report_sim/Kinematics/Kinematics 313/s_312 - A ==
  s : Inport
  Demux : Demux  Outputs=3
  Product : Product  Inputs=3  Multiplication=Matrix(*)
  R1 : Subsystem
  R2 : Subsystem
  R3 : Subsystem
  A : Outport
  wires:
  s/1 -> Demux/1  "s"
  R1/1(R1) -> Product/2
  R3/1(R3) -> Product/3
  R2/1(R2) -> Product/1
  Product/1 -> A/1
  Demux/2 -> R1/1(x)  "theta"
  Demux/1 -> R3/1(x)  "phi"
  Demux/3 -> R2/1(x)  "psi"

== system disturbances_report_sim/Kinematics/Kinematics 313/s_313 - A ==
  s : Inport
  Demux : Demux  Outputs=3
  Product : Product  Inputs=3  Multiplication=Matrix(*)
  R1 : Subsystem
  R3_1 : Subsystem
  R3_2 : Subsystem
  A : Outport
  wires:
  Demux/3 -> R3_2/1(x)  "psi"
  Demux/1 -> R3_1/1(x)  "phi"
  Demux/2 -> R1/1(x)  "theta"
  Product/1 -> A/1
  R1/1(R1) -> Product/2
  s/1 -> Demux/1  "s"
  R3_1/1(R3) -> Product/3
  R3_2/1(R3) -> Product/1

== system disturbances_report_sim/SRP torque/SRP forces calc/shadow check ==
  In1 : Inport
  Compare To Constant : simulink/Logic and Bit Operations/Compare To Constant  relop=<  const=0  OutDataTypeStr=boolean
  Product5 : Product
  Out1 : Outport
  wires:
  Product5/1 -> Out1/1
  In1/1 -> Compare To Constant/1, Product5/1
  Compare To Constant/1 -> Product5/2

== system disturbances_report_sim/Subsystem/Magnetic Field/R_en ==
  Clock : Clock
  Constant : Constant  Value=omegaE
  Constant1 : Constant  Value=[0; 0; 1]
  Constant2 : Constant  Value=0
  Cos : Trigonometry  Operator=cos
  Gain : Gain  Gain=-1
  Matrix Concatenate : Concatenate  NumInputs=3  Mode=Multidimensional array  ConcatenateDimension=2
  Product : Product
  Sin : Trigonometry
  Vector Concatenate : Concatenate  NumInputs=3
  Vector Concatenate1 : Concatenate  NumInputs=3
  R_en : Outport
  wires:
  Clock/1 -> Product/1
  Constant/1 -> Product/2
  Product/1 -> Cos/1, Sin/1
  Vector Concatenate/1 -> Matrix Concatenate/1
  Vector Concatenate1/1 -> Matrix Concatenate/2
  Cos/1 -> Vector Concatenate1/2, Vector Concatenate/1
  Constant1/1 -> Matrix Concatenate/3
  Gain/1 -> Vector Concatenate/2
  Sin/1 -> Vector Concatenate1/1, Gain/1
  Constant2/1 -> Vector Concatenate1/3, Vector Concatenate/3
  Matrix Concatenate/1 -> R_en/1

== system disturbances_report_sim/Kinematics/Kinematics 312/Euler angles/Subsystem ==
  In1 : Inport
  In2 : Inport  Port=2
  In3 : Inport  Port=3
  Cos : Trigonometry  Operator=cos
  Product : Product
  Product1 : Product
  Sin : Trigonometry
  Sum : Sum
  Out1 : Outport
  wires:
  In3/1 -> Sin/1, Cos/1
  In1/1 -> Product/1
  Cos/1 -> Product/2
  Sin/1 -> Product1/1
  In2/1 -> Product1/2
  Product/1 -> Sum/1
  Product1/1 -> Sum/2
  Sum/1 -> Out1/1

== system disturbances_report_sim/Kinematics/Kinematics 312/Euler angles/Subsystem1 ==
  In1 : Inport
  In2 : Inport  Port=2
  In3 : Inport  Port=3
  Cos : Trigonometry  Operator=cos
  Product : Product
  Product1 : Product
  Sin : Trigonometry
  Sum : Sum
  Out1 : Outport
  wires:
  Sum/1 -> Out1/1
  Product1/1 -> Sum/2
  Product/1 -> Sum/1
  In2/1 -> Product1/2
  Sin/1 -> Product1/1
  Cos/1 -> Product/2
  In1/1 -> Product/1
  In3/1 -> Cos/1, Sin/1

== system disturbances_report_sim/Kinematics/Kinematics 312/Euler angles/Subsystem2 ==
  In1 : Inport
  In2 : Inport  Port=2
  In3 : Inport  Port=3
  Cos : Trigonometry  Operator=cos
  Product : Product
  Product1 : Product
  Sin : Trigonometry
  Sum : Sum
  Out1 : Outport
  wires:
  In3/1 -> Sin/1, Cos/1
  In1/1 -> Product/1
  Cos/1 -> Product/2
  Sin/1 -> Product1/1
  In2/1 -> Product1/2
  Product/1 -> Sum/1
  Product1/1 -> Sum/2
  Sum/1 -> Out1/1

== system disturbances_report_sim/Kinematics/Kinematics 312/s_312 - A/R1 ==
  x : Inport
  Constant : Constant  Value=[1; 0; 0]
  Constant1 : Constant  Value=0
  Cos : Trigonometry  Operator=cos
  Gain : Gain  Gain=-1
  Matrix Concatenate : Concatenate  NumInputs=3  Mode=Multidimensional array  ConcatenateDimension=2
  Sin : Trigonometry
  Vector Concatenate : Concatenate  NumInputs=3
  Vector Concatenate1 : Concatenate  NumInputs=3
  R1 : Outport
  wires:
  Matrix Concatenate/1 -> R1/1
  x/1 -> Cos/1, Sin/1
  Vector Concatenate1/1 -> Matrix Concatenate/2
  Constant/1 -> Matrix Concatenate/1
  Vector Concatenate/1 -> Matrix Concatenate/3
  Constant1/1 -> Vector Concatenate/1, Vector Concatenate1/1
  Cos/1 -> Vector Concatenate/3, Vector Concatenate1/2
  Gain/1 -> Vector Concatenate1/3
  Sin/1 -> Vector Concatenate/2, Gain/1

== system disturbances_report_sim/Kinematics/Kinematics 312/s_312 - A/R2 ==
  x : Inport
  Constant : Constant  Value=[0; 1; 0]
  Constant1 : Constant  Value=0
  Cos : Trigonometry  Operator=cos
  Gain : Gain  Gain=-1
  Matrix Concatenate : Concatenate  NumInputs=3  Mode=Multidimensional array  ConcatenateDimension=2
  Sin : Trigonometry
  Vector Concatenate : Concatenate  NumInputs=3
  Vector Concatenate1 : Concatenate  NumInputs=3
  R2 : Outport
  wires:
  Vector Concatenate/1 -> Matrix Concatenate/1
  x/1 -> Sin/1, Cos/1
  Matrix Concatenate/1 -> R2/1
  Constant/1 -> Matrix Concatenate/2
  Vector Concatenate1/1 -> Matrix Concatenate/3
  Constant1/1 -> Vector Concatenate/2, Vector Concatenate1/2
  Cos/1 -> Vector Concatenate1/3, Vector Concatenate/1
  Sin/1 -> Gain/1, Vector Concatenate/3
  Gain/1 -> Vector Concatenate1/1

== system disturbances_report_sim/Kinematics/Kinematics 312/s_312 - A/R3 ==
  x : Inport
  Constant : Constant  Value=[0; 0; 1]
  Constant1 : Constant  Value=0
  Cos : Trigonometry  Operator=cos
  Gain : Gain  Gain=-1
  Matrix Concatenate : Concatenate  NumInputs=3  Mode=Multidimensional array  ConcatenateDimension=2
  Sin : Trigonometry
  Vector Concatenate : Concatenate  NumInputs=3
  Vector Concatenate1 : Concatenate  NumInputs=3
  R3 : Outport
  wires:
  Vector Concatenate/1 -> Matrix Concatenate/1
  Sin/1 -> Vector Concatenate1/1, Gain/1
  Cos/1 -> Vector Concatenate1/2, Vector Concatenate/1
  Constant/1 -> Matrix Concatenate/3
  Gain/1 -> Vector Concatenate/2
  Vector Concatenate1/1 -> Matrix Concatenate/2
  x/1 -> Sin/1, Cos/1
  Constant1/1 -> Vector Concatenate/3, Vector Concatenate1/3
  Matrix Concatenate/1 -> R3/1

== system disturbances_report_sim/Kinematics/Kinematics 312/s_313 - A/R1 ==
  x : Inport
  Constant : Constant  Value=[1; 0; 0]
  Constant1 : Constant  Value=0
  Cos : Trigonometry  Operator=cos
  Gain : Gain  Gain=-1
  Matrix Concatenate : Concatenate  NumInputs=3  Mode=Multidimensional array  ConcatenateDimension=2
  Sin : Trigonometry
  Vector Concatenate : Concatenate  NumInputs=3
  Vector Concatenate1 : Concatenate  NumInputs=3
  R1 : Outport
  wires:
  Sin/1 -> Gain/1, Vector Concatenate/2
  Gain/1 -> Vector Concatenate1/3
  Cos/1 -> Vector Concatenate1/2, Vector Concatenate/3
  Constant1/1 -> Vector Concatenate1/1, Vector Concatenate/1
  Vector Concatenate/1 -> Matrix Concatenate/3
  Constant/1 -> Matrix Concatenate/1
  Vector Concatenate1/1 -> Matrix Concatenate/2
  x/1 -> Sin/1, Cos/1
  Matrix Concatenate/1 -> R1/1

== system disturbances_report_sim/Kinematics/Kinematics 312/s_313 - A/R3_1 ==
  x : Inport
  Constant : Constant  Value=[0; 0; 1]
  Constant1 : Constant  Value=0
  Cos : Trigonometry  Operator=cos
  Gain : Gain  Gain=-1
  Matrix Concatenate : Concatenate  NumInputs=3  Mode=Multidimensional array  ConcatenateDimension=2
  Sin : Trigonometry
  Vector Concatenate : Concatenate  NumInputs=3
  Vector Concatenate1 : Concatenate  NumInputs=3
  R3 : Outport
  wires:
  Matrix Concatenate/1 -> R3/1
  Constant1/1 -> Vector Concatenate1/3, Vector Concatenate/3
  x/1 -> Cos/1, Sin/1
  Vector Concatenate1/1 -> Matrix Concatenate/2
  Gain/1 -> Vector Concatenate/2
  Constant/1 -> Matrix Concatenate/3
  Cos/1 -> Vector Concatenate/1, Vector Concatenate1/2
  Sin/1 -> Gain/1, Vector Concatenate1/1
  Vector Concatenate/1 -> Matrix Concatenate/1

== system disturbances_report_sim/Kinematics/Kinematics 312/s_313 - A/R3_2 ==
  x : Inport
  Constant : Constant  Value=[0; 0; 1]
  Constant1 : Constant  Value=0
  Cos : Trigonometry  Operator=cos
  Gain : Gain  Gain=-1
  Matrix Concatenate : Concatenate  NumInputs=3  Mode=Multidimensional array  ConcatenateDimension=2
  Sin : Trigonometry
  Vector Concatenate : Concatenate  NumInputs=3
  Vector Concatenate1 : Concatenate  NumInputs=3
  R3 : Outport
  wires:
  Vector Concatenate/1 -> Matrix Concatenate/1
  Sin/1 -> Vector Concatenate1/1, Gain/1
  Cos/1 -> Vector Concatenate1/2, Vector Concatenate/1
  Constant/1 -> Matrix Concatenate/3
  Gain/1 -> Vector Concatenate/2
  Vector Concatenate1/1 -> Matrix Concatenate/2
  x/1 -> Sin/1, Cos/1
  Constant1/1 -> Vector Concatenate/3, Vector Concatenate1/3
  Matrix Concatenate/1 -> R3/1

== system disturbances_report_sim/Kinematics/Kinematics 313/Euler angles/Subsystem ==
  In1 : Inport
  In2 : Inport  Port=2
  In3 : Inport  Port=3
  Cos : Trigonometry  Operator=cos
  Product : Product
  Product1 : Product
  Sin : Trigonometry
  Sum : Sum
  Out1 : Outport
  wires:
  Sum/1 -> Out1/1
  Product1/1 -> Sum/2
  Product/1 -> Sum/1
  In2/1 -> Product1/2
  Sin/1 -> Product1/1
  Cos/1 -> Product/2
  In1/1 -> Product/1
  In3/1 -> Cos/1, Sin/1

== system disturbances_report_sim/Kinematics/Kinematics 313/Euler angles/Subsystem1 ==
  In1 : Inport
  In2 : Inport  Port=2
  In3 : Inport  Port=3
  Cos : Trigonometry  Operator=cos
  Product : Product
  Product1 : Product
  Sin : Trigonometry
  Sum : Sum
  Out1 : Outport
  wires:
  In3/1 -> Sin/1, Cos/1
  In1/1 -> Product/1
  Cos/1 -> Product/2
  Sin/1 -> Product1/1
  In2/1 -> Product1/2
  Product/1 -> Sum/1
  Product1/1 -> Sum/2
  Sum/1 -> Out1/1

== system disturbances_report_sim/Kinematics/Kinematics 313/Euler angles/Subsystem2 ==
  In1 : Inport
  In2 : Inport  Port=2
  In3 : Inport  Port=3
  Cos : Trigonometry  Operator=cos
  Product : Product
  Product1 : Product
  Sin : Trigonometry
  Sum : Sum
  Out1 : Outport
  wires:
  Sum/1 -> Out1/1
  Product1/1 -> Sum/2
  Product/1 -> Sum/1
  In2/1 -> Product1/2
  Sin/1 -> Product1/1
  Cos/1 -> Product/2
  In1/1 -> Product/1
  In3/1 -> Cos/1, Sin/1

== system disturbances_report_sim/Kinematics/Kinematics 313/s_312 - A/R1 ==
  x : Inport
  Constant : Constant  Value=[1; 0; 0]
  Constant1 : Constant  Value=0
  Cos : Trigonometry  Operator=cos
  Gain : Gain  Gain=-1
  Matrix Concatenate : Concatenate  NumInputs=3  Mode=Multidimensional array  ConcatenateDimension=2
  Sin : Trigonometry
  Vector Concatenate : Concatenate  NumInputs=3
  Vector Concatenate1 : Concatenate  NumInputs=3
  R1 : Outport
  wires:
  Matrix Concatenate/1 -> R1/1
  x/1 -> Cos/1, Sin/1
  Vector Concatenate1/1 -> Matrix Concatenate/2
  Constant/1 -> Matrix Concatenate/1
  Vector Concatenate/1 -> Matrix Concatenate/3
  Constant1/1 -> Vector Concatenate/1, Vector Concatenate1/1
  Cos/1 -> Vector Concatenate/3, Vector Concatenate1/2
  Gain/1 -> Vector Concatenate1/3
  Sin/1 -> Vector Concatenate/2, Gain/1

== system disturbances_report_sim/Kinematics/Kinematics 313/s_312 - A/R2 ==
  x : Inport
  Constant : Constant  Value=[0; 1; 0]
  Constant1 : Constant  Value=0
  Cos : Trigonometry  Operator=cos
  Gain : Gain  Gain=-1
  Matrix Concatenate : Concatenate  NumInputs=3  Mode=Multidimensional array  ConcatenateDimension=2
  Sin : Trigonometry
  Vector Concatenate : Concatenate  NumInputs=3
  Vector Concatenate1 : Concatenate  NumInputs=3
  R2 : Outport
  wires:
  Vector Concatenate/1 -> Matrix Concatenate/1
  x/1 -> Sin/1, Cos/1
  Matrix Concatenate/1 -> R2/1
  Constant/1 -> Matrix Concatenate/2
  Vector Concatenate1/1 -> Matrix Concatenate/3
  Constant1/1 -> Vector Concatenate/2, Vector Concatenate1/2
  Cos/1 -> Vector Concatenate1/3, Vector Concatenate/1
  Sin/1 -> Gain/1, Vector Concatenate/3
  Gain/1 -> Vector Concatenate1/1

== system disturbances_report_sim/Kinematics/Kinematics 313/s_312 - A/R3 ==
  x : Inport
  Constant : Constant  Value=[0; 0; 1]
  Constant1 : Constant  Value=0
  Cos : Trigonometry  Operator=cos
  Gain : Gain  Gain=-1
  Matrix Concatenate : Concatenate  NumInputs=3  Mode=Multidimensional array  ConcatenateDimension=2
  Sin : Trigonometry
  Vector Concatenate : Concatenate  NumInputs=3
  Vector Concatenate1 : Concatenate  NumInputs=3
  R3 : Outport
  wires:
  Vector Concatenate/1 -> Matrix Concatenate/1
  Sin/1 -> Vector Concatenate1/1, Gain/1
  Cos/1 -> Vector Concatenate1/2, Vector Concatenate/1
  Constant/1 -> Matrix Concatenate/3
  Gain/1 -> Vector Concatenate/2
  Vector Concatenate1/1 -> Matrix Concatenate/2
  x/1 -> Sin/1, Cos/1
  Constant1/1 -> Vector Concatenate/3, Vector Concatenate1/3
  Matrix Concatenate/1 -> R3/1
